simulink model "xieboduoji_13fangzhennow"  (R2023a)
settings: Solver=ode4  StartTime=0.0  StopTime=2.2  FixedStep=5e-7  RelTol=1e-3
undefined symbols (not defined in the file or in its folder): magnitude
libraries: simulink x417, spsRMSLib x70, spsCurrentMeasurementLib x32, spsVoltageMeasurementLib x31, powerlib_meascontrol x24, spsFourierLib x21, spsGroundLib x19, spsThreePhasePISectionLineLib x17, spsThreePhaseSeriesRLCBranchLib x14, spsdq0toAlphaBetaZeroLib x13, spsSeriesRLCBranchLib x11, spsUniversalBridgeLib x11
(part 4 of 12)

== system xieboduoji_13fangzhennow/node14/PV15kW3/Subsystem9 ==
  di : Inport
  Enable : EnablePort
  Pulse tor2 : DiscretePulseGenerator  PulseType=Time based  Period=10e-5  PulseWidth=50
  "integral " : Subsystem  TreatAsAtomicUnit=on
  w : Outport
  wires:
  Pulse tor2/1 -> "integral "/Trigger
  di/1 -> "integral "/1(di)
  "integral "/1(w) -> w/1

== system xieboduoji_13fangzhennow/node14/PV15kW3/改进PLL1 ==
  abc : Inport
  Add : Sum
  Alpha-Beta-Zero to dq0 : spsAlphaBetaZerotodq0Lib/Alpha-Beta-Zero to dq0  Alignment=Aligned with phase A axis
  Constant : Constant  Value=100*pi
  Constant3 : Constant  Value=2*pi
  Demux1 : Demux  Outputs=3
  Gain1 : Gain  Commented=on  Gain=0.5/pi
  Goto2 : Goto  Commented=on  GotoTag=vp
  Integrator : Integrator
  Math Function : Math  Operator=mod  SignedPower=on
  PI : Subsystem  TreatAsAtomicUnit=on
  PID Controller : slpidlib/PID Controller  Controller=P  Form=Parallel  TimeDomain=Discrete-time  UseExternalTs=off  SampleTime=10e-5  IntegratorMethod=Forward Euler  FilterMethod=Forward Euler  ControllerParametersSource=internal  P=1  I=1  UseKiTs=off  D=0  N=100  UseFilter=on  TunerSelectOption=Transfer Function Based (PID Tuner App)  InitialConditionSource=internal  InitialConditionForIntegrator=0  InitialConditionForFilter=0  DifferentiatorICPrevScaledInput=0  ExternalReset=none  TrackingMode=off  Kt=1  LimitOutput=off  SatLimitsSource=internal  UpperSaturationLimit=inf  LowerSaturationLimit=-inf  LinearizeAsGain=on  AntiWindupMode=none  Kb=1  LimitIntegrator=off  UpperIntegratorSaturationLimit=inf  LowerIntegratorSaturationLimit=-inf  POutMin=[]  POutMax=[]  IOutMin=[]  IOutMax=[]  DOutMin=[]  DOutMax=[]  NOutMin=[]  NOutMax=[]  SumOutMin=[]  SumOutMax=[]  SaturationOutMin=[]  SaturationOutMax=[]  PParamMin=[]  PParamMax=[]  IParamMin=[]  IParamMax=[]  DParamMin=[]  DParamMax=[]  NParamMin=[]  NParamMax=[]  KbParamMin=[]  KbParamMax=[]  KtParamMin=[]  KtParamMax=[]  KbOutMin=[]  KbOutMax=[]  KtOutMin=[]  KtOutMax=[]  IntegratorOutMin=[]  IntegratorOutMax=[]  FilterOutMin=[]  FilterOutMax=[]  SumI1OutMin=[]  SumI1OutMax=[]  SumI2OutMin=[]  SumI2OutMax=[]  SumI3OutMin=[]  SumI3OutMax=[]  SumI4OutMin=[]  SumI4OutMax=[]  SumDOutMin=[]  SumDOutMax=[]  DifferentiatorOutMin=[]  DifferentiatorOutMax=[]  FilterDiffOutCoefMin=[]  FilterDiffOutCoefMax=[]  ReciprocalOutMin=[]  ReciprocalOutMax=[]  SumDenOutMin=[]  SumDenOutMax=[]  SumNumOutMin=[]  SumNumOutMax=[]  DivideOutMin=[]  DivideOutMax=[]  UdiffTsProdOutMin=[]  UdiffTsProdOutMax=[]  NTsProdOutMin=[]  NTsProdOutMax=[]  UintegralTsProdOutMin=[]  UintegralTsProdOutMax=[]  UngainTsProdOutMin=[]  UngainTsProdOutMax=[]  ClampingZeroOutDataTypeStr=Inherit: Inherit via back propagation  ClampingZeroOutMin=[]  ClampingZeroOutMax=[]  FilterDenConstantOutDataTypeStr=Inherit: Inherit via back propagation  FilterDenConstantOutMin=[]  FilterDenConstantOutMax=[]  PCopyOutDataTypeStr=Inherit: Inherit via back propagation  PCopyOutMin=[]  PCopyOutMax=[]  NCopyOutDataTypeStr=Inherit: Inherit via back propagation  NCopyOutMin=[]  NCopyOutMax=[]  IntegratorContinuousStateAttributes=''  IntegratorStateMustResolveToSignalObject=off  IntegratorRTWStateStorageClass=Auto  FilterContinuousStateAttributes=''  FilterStateMustResolveToSignalObject=off  FilterRTWStateStorageClass=Auto  ParallelPVariant=InternalParameters  IdealPVariant=Disabled  IVariant=Disabled  DVariant=Disabled  IntegratorVariant=Disabled  SatVariant=Disabled  AWVariant=Disabled  PCopyVariant=Disabled  TRVariant=Disabled  FdbkBlocksVariant=Forward  IdealPFdbkVariant=Disabled  SatFdbkVariant=Disabled  DerivativeFilterVariant=Disabled  NVariant=Disabled  NCopyVariant=Disabled_SignalSpec  FilterICVariant=Disabled  IntegratorICVariant=Disabled  ExternalResetVariant=Disabled  TRSumVariant=Passthrough  SumFdbkVariant=Disabled  SumVariant=Passthrough_P  TsampFilterVariant=InternalTs  TsampNgainVariant=Passthrough  TsampIntegralVariant=Disabled_SignalSpec  ExternalSaturationOutDataTypeStr=Inherit: Same as second input
  Pulse tor2 : DiscretePulseGenerator  PulseType=Time based  Period=5e-5  PulseWidth=50
  Scope : Scope
  Scope1 : Scope  Commented=on
  Scope3 : Scope  Commented=on
  Subsystem2 : Subsystem
  Terminator : Terminator
  abc to Alpha-Beta-Zero1 : spsabctoAlphaBetaZeroLib/abc to Alpha-Beta-Zero
  mean1 : spsMeanLib/Mean  Commented=on  Freq=100  Vinit=0  Ts=10e-5
  mean2 : spsMeanLib/Mean  Freq=100  Vinit=0  Ts=10e-5
  Out2 : Outport
  vab0 : Outport  Port=2
  wires:
  Demux1/3 -> Terminator/1
  mean2/1 -> PID Controller/1, PI/1(Vgq)
  abc/1 -> abc to Alpha-Beta-Zero1/1
  mean1/1 -> Scope3/1, Goto2/1
  Demux1/2 -> mean2/1
  Pulse tor2/1 -> PI/Trigger
  PI/1(w) -> Add/2
  Constant/1 -> Add/1
  Alpha-Beta-Zero to dq0/1 -> Demux1/1
  Add/1 -> Gain1/1, Integrator/1
  Math Function/1 -> Out2/1, [wt], Alpha-Beta-Zero to dq0/2
  Constant3/1 -> Math Function/2
  Integrator/1 -> Math Function/1
  Gain1/1 -> Scope1/1
  PID Controller/1 -> Scope/1
  Demux1/1 -> mean1/1
  abc to Alpha-Beta-Zero1/1 -> vab0/1, Subsystem2/1(In1)
  Subsystem2/1(Out1) -> Alpha-Beta-Zero to dq0/1

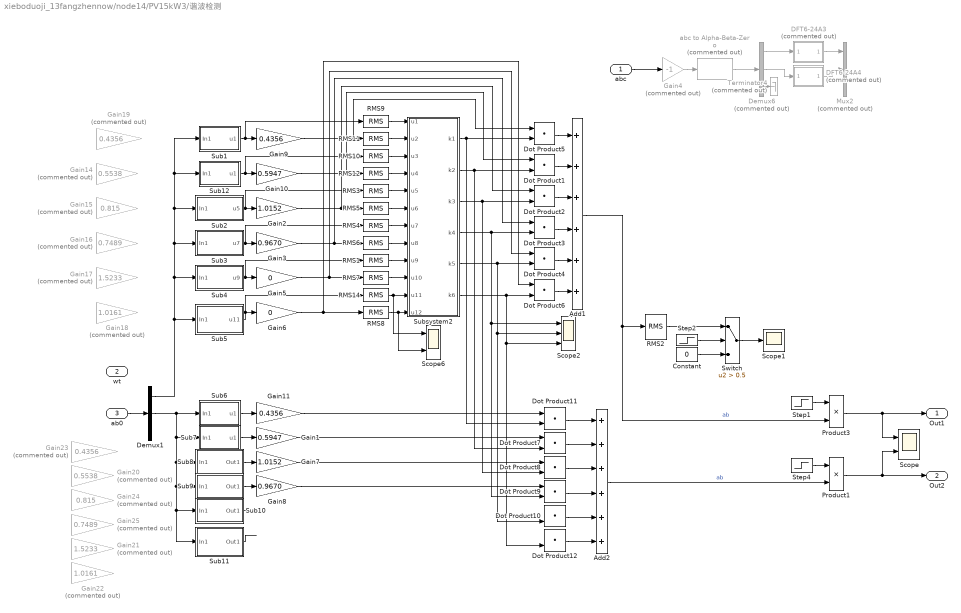
== system xieboduoji_13fangzhennow/node14/PV15kW3/谐波检测 ==
  abc : Inport
  wt : Inport  Port=2
  ab0 : Inport  Port=3
  Add1 : Sum  Inputs=++++++
  Add2 : Sum  Inputs=++++++
  Constant : Constant  Value=0
  DFT6-24A3 : Subsystem  Commented=on
  DFT6-24A4 : Subsystem  Commented=on
  Demux1 : Demux  Outputs=3
  Demux6 : Demux  Commented=on  Outputs=3
  Dot Product{1..12} (12 alike) : DotProduct  OutDataTypeStr=Inherit: Inherit via internal rule
  Gain1 : Gain  Gain=0.5947
  Gain10 : Gain  Gain=0.5947
  Gain11 : Gain  Gain=0.4356
  Gain14 : Gain  Commented=on  Gain=0.5538
  Gain15 : Gain  Commented=on  Gain=0.815
  Gain16 : Gain  Commented=on  Gain=0.7489
  Gain17 : Gain  Commented=on  Gain=1.5233
  Gain18 : Gain  Commented=on  Gain=1.0161
  Gain19 : Gain  Commented=on  Gain=0.4356
  Gain2 : Gain  Gain=1.0152
  Gain20 : Gain  Commented=on  Gain=0.5538
  Gain21 : Gain  Commented=on  Gain=1.5233
  Gain22 : Gain  Commented=on  Gain=1.0161
  Gain23 : Gain  Commented=on  Gain=0.4356
  Gain24 : Gain  Commented=on  Gain=0.815
  Gain25 : Gain  Commented=on  Gain=0.7489
  Gain3 : Gain  Gain=0.9670
  Gain4 : Gain  Commented=on  Gain=-1
  Gain5 : Gain  Gain=0
  Gain6 : Gain  Gain=0
  Gain7 : Gain  Gain=1.0152
  Gain8 : Gain  Gain=0.9670
  Gain9 : Gain  Gain=0.4356
  Mux2 : Mux  Commented=on  Inputs=3
  Product1 : Product
  Product3 : Product
  RMS{1,3..12,14} (12 alike) : spsRMSLib/RMS  TrueRMS=on  Freq=100  RMSInit=0  Ts=5e-5
  RMS2 : spsRMSLib/RMS  TrueRMS=on  Freq=50  RMSInit=0  Ts=5e-5
  Scope : Scope  NumInputPorts=2
  Scope1 : Scope
  Scope2 : Scope  NumInputPorts=3
  Scope6 : Scope  NumInputPorts=2
  Step1 : Step  After=-1  SampleTime=0
  Step2 : Step  SampleTime=0
  Step4 : Step  After=-1  SampleTime=0
  Sub1 : Subsystem
  Sub10 : Subsystem
  Sub11 : Subsystem
  Sub12 : Subsystem
  Sub2 : Subsystem
  Sub3 : Subsystem
  Sub4 : Subsystem
  Sub5 : Subsystem
  Sub6 : Subsystem
  Sub7 : Subsystem
  Sub8 : Subsystem
  Sub9 : Subsystem
  Subsystem2 : Subsystem
  Switch : Switch  Criteria=u2 > Threshold  Threshold=0.5  SaturateOnIntegerOverflow=off  InputSameDT=off
  Terminator4 : Terminator  Commented=on
  abc to Alpha-Beta-Zero : spsabctoAlphaBetaZeroLib/abc to Alpha-Beta-Zero  Commented=on
  Out1 : Outport
  Out2 : Outport  Port=2
  wires:
  abc/1 -> Gain4/1
  Step1/1 -> Product3/1
  abc to Alpha-Beta-Zero/1 -> Demux6/1
  DFT6-24A4/1(Out1) -> Mux2/2
  DFT6-24A3/1(Out1) -> Mux2/1
  Demux6/2 -> DFT6-24A4/1(In1)
  Demux6/1 -> DFT6-24A3/1(In1)
  Demux6/3 -> Terminator4/1
  ab0/1 -> Demux1/1
  Step2/1 -> Switch/2
  Constant/1 -> Switch/3
  Switch/1 -> Scope1/1
  Gain4/1 -> abc to Alpha-Beta-Zero/1
  Sub5/1(u11) -> RMS14/1, Gain6/1
  Sub4/1(u9) -> Gain5/1, RMS1/1
  Sub3/1(u7) -> RMS4/1, Gain3/1
  Sub2/1(u5) -> RMS3/1, Gain2/1
  Demux1/1 -> Sub12/1(In1), Sub1/1(In1), Sub2/1(In1), Sub3/1(In1), Sub4/1(In1), Sub5/1(In1)
  Sub12/1(u1) -> RMS10/1, Gain10/1
  Sub1/1(u1) -> RMS9/1, Gain9/1
  Subsystem2/1(k1) -> Dot Product11/2, Dot Product5/2
  Subsystem2/2(k2) -> Dot Product7/2, Dot Product1/2
  Subsystem2/3(k3) -> Dot Product8/2, Dot Product2/2
  Subsystem2/4(k4) -> Scope2/1, Dot Product9/2, Dot Product3/2
  Subsystem2/5(k5) -> Dot Product10/2, Scope2/2, Dot Product4/2
  Add1/1 -> Product3/2, RMS2/1  "ab"
  Sub6/1(u1) -> Gain11/1
  Sub7/1(u1) -> Gain1/1
  Sub8/1(Out1) -> Gain7/1
  Sub9/1(Out1) -> Gain8/1
  Sub10/1(Out1) -> ?
  Sub11/1(Out1) -> ?
  Demux1/2 -> Sub6/1(In1), Sub7/1(In1), Sub11/1(In1), Sub10/1(In1), Sub9/1(In1), Sub8/1(In1)
  Dot Product12/1 -> Add2/6
  Dot Product10/1 -> Add2/5
  Gain9/1 -> RMS11/1, Dot Product5/1
  Gain2/1 -> RMS5/1, Dot Product2/1
  Gain3/1 -> Dot Product3/1, RMS6/1
  Gain5/1 -> RMS7/1, Dot Product4/1
  Gain6/1 -> Dot Product6/1, RMS8/1
  Gain11/1 -> Dot Product11/1
  Gain1/1 -> Dot Product7/1
  Gain7/1 -> Dot Product8/1
  Gain8/1 -> Dot Product9/1
  ? -> Dot Product10/1
  ? -> Dot Product12/1
  RMS2/1 -> Switch/1
  RMS7/1 -> Subsystem2/10(u10)
  RMS8/1 -> Scope6/2, Subsystem2/12(u12)
  Gain10/1 -> RMS12/1, Dot Product1/1
  RMS9/1 -> Subsystem2/1(u1)
  RMS1/1 -> Subsystem2/9(u9)
  RMS14/1 -> Subsystem2/11(u11), Scope6/1
  Dot Product6/1 -> Add1/6
  Dot Product4/1 -> Add1/5
  RMS11/1 -> Subsystem2/2(u2)
  RMS10/1 -> Subsystem2/3(u3)
  RMS12/1 -> Subsystem2/4(u4)
  RMS3/1 -> Subsystem2/5(u5)
  RMS5/1 -> Subsystem2/6(u6)
  RMS4/1 -> Subsystem2/7(u7)
  RMS6/1 -> Subsystem2/8(u8)
  Add2/1 -> Product1/2  "ab"
  Step4/1 -> Product1/1
  Product1/1 -> Scope/2, Out2/1
  Product3/1 -> Scope/1, Out1/1
  Dot Product5/1 -> Add1/1
  Dot Product1/1 -> Add1/2
  Dot Product2/1 -> Add1/3
  Dot Product3/1 -> Add1/4
  Subsystem2/6(k6) -> Scope2/3, Dot Product12/2, Dot Product6/2
  Dot Product11/1 -> Add2/1
  Dot Product7/1 -> Add2/2
  Dot Product8/1 -> Add2/3
  Dot Product9/1 -> Add2/4

== system xieboduoji_13fangzhennow/node14/Subsystem1/RMS1 ==
  u1 : Inport
  u3 : Inport  Port=2
  u4 : Inport  Port=3
  u5 : Inport  Port=4
  u6 : Inport  Port=5
  u2 : Inport  Port=6
  Trigger : TriggerPort  VariantControl=(inherit)
  Scope : Scope  Commented=on
  Scope1 : Scope  Commented=on
  xunidiandao : MATLAB Function  TreatAsAtomicUnit=on
  k1 : Outport  VectorParamsAs1DForOutWhenUnconnected=off
  k2 : Outport  Port=2  VectorParamsAs1DForOutWhenUnconnected=off
  k3 : Outport  Port=3  VectorParamsAs1DForOutWhenUnconnected=off
  k4 : Outport  Port=4  VectorParamsAs1DForOutWhenUnconnected=off
  k5 : Outport  Port=5  VectorParamsAs1DForOutWhenUnconnected=off
  k6 : Outport  Port=6  VectorParamsAs1DForOutWhenUnconnected=off
  k7 : Outport  Port=7  VectorParamsAs1DForOutWhenUnconnected=off
  k8 : Outport  Port=8  VectorParamsAs1DForOutWhenUnconnected=off
  k9 : Outport  Port=9  VectorParamsAs1DForOutWhenUnconnected=off
  k10 : Outport  Port=10  VectorParamsAs1DForOutWhenUnconnected=off
  k11 : Outport  Port=11  VectorParamsAs1DForOutWhenUnconnected=off
  k12 : Outport  Port=12  VectorParamsAs1DForOutWhenUnconnected=off
  wires:
  xunidiandao/13(x) -> Scope/1
  u3/1 -> xunidiandao/2(u2)
  u4/1 -> xunidiandao/3(u3)
  u5/1 -> xunidiandao/4(u4)
  u6/1 -> xunidiandao/5(u5)
  u2/1 -> xunidiandao/6(u6)
  u1/1 -> xunidiandao/1(u1)
  xunidiandao/12(y66) -> k12/1
  xunidiandao/11(y6) -> k11/1
  xunidiandao/10(y55) -> k10/1
  xunidiandao/9(y5) -> k9/1
  xunidiandao/8(y44) -> k8/1
  xunidiandao/7(y4) -> k7/1
  xunidiandao/6(y33) -> k6/1
  xunidiandao/5(y3) -> k5/1
  xunidiandao/4(y22) -> k4/1
  xunidiandao/3(y2) -> k3/1
  xunidiandao/2(y11) -> k2/1
  xunidiandao/1(y1) -> k1/1, Scope1/1

== system xieboduoji_13fangzhennow/node14/Subsystem2/RMS1 ==
  u1 : Inport
  u3 : Inport  Port=2
  u4 : Inport  Port=3
  u5 : Inport  Port=4
  u6 : Inport  Port=5
  u2 : Inport  Port=6
  Trigger : TriggerPort  VariantControl=(inherit)
  Scope : Scope  Commented=on
  Scope1 : Scope  Commented=on
  xunidiandao : MATLAB Function  TreatAsAtomicUnit=on
  k1 : Outport  VectorParamsAs1DForOutWhenUnconnected=off
  k2 : Outport  Port=2  VectorParamsAs1DForOutWhenUnconnected=off
  k3 : Outport  Port=3  VectorParamsAs1DForOutWhenUnconnected=off
  k4 : Outport  Port=4  VectorParamsAs1DForOutWhenUnconnected=off
  k5 : Outport  Port=5  VectorParamsAs1DForOutWhenUnconnected=off
  k6 : Outport  Port=6  VectorParamsAs1DForOutWhenUnconnected=off
  k7 : Outport  Port=7  VectorParamsAs1DForOutWhenUnconnected=off
  k8 : Outport  Port=8  VectorParamsAs1DForOutWhenUnconnected=off
  k9 : Outport  Port=9  VectorParamsAs1DForOutWhenUnconnected=off
  k10 : Outport  Port=10  VectorParamsAs1DForOutWhenUnconnected=off
  k11 : Outport  Port=11  VectorParamsAs1DForOutWhenUnconnected=off
  k12 : Outport  Port=12  VectorParamsAs1DForOutWhenUnconnected=off
  wires:
  xunidiandao/1(y1) -> Scope1/1, k1/1
  xunidiandao/2(y11) -> k2/1
  xunidiandao/3(y2) -> k3/1
  xunidiandao/4(y22) -> k4/1
  xunidiandao/5(y3) -> k5/1
  xunidiandao/6(y33) -> k6/1
  xunidiandao/7(y4) -> k7/1
  xunidiandao/8(y44) -> k8/1
  xunidiandao/9(y5) -> k9/1
  xunidiandao/10(y55) -> k10/1
  xunidiandao/11(y6) -> k11/1
  xunidiandao/12(y66) -> k12/1
  u1/1 -> xunidiandao/1(u1)
  u2/1 -> xunidiandao/6(u6)
  u6/1 -> xunidiandao/5(u5)
  u5/1 -> xunidiandao/4(u4)
  u4/1 -> xunidiandao/3(u3)
  u3/1 -> xunidiandao/2(u2)
  xunidiandao/13(x) -> Scope/1

== system xieboduoji_13fangzhennow/node14/谐波源/Subsystem1 ==
  u1 : Inport
  u3 : Inport  Port=2
  u4 : Inport  Port=3
  u5 : Inport  Port=4
  u6 : Inport  Port=5
  u2 : Inport  Port=6
  Pul : DiscretePulseGenerator  PulseType=Time based  Period=5e-5  PulseWidth=40
  RMS1 : Subsystem  TreatAsAtomicUnit=on
  k1 : Outport  VectorParamsAs1DForOutWhenUnconnected=off
  k2 : Outport  Port=2  VectorParamsAs1DForOutWhenUnconnected=off
  k3 : Outport  Port=3  VectorParamsAs1DForOutWhenUnconnected=off
  k4 : Outport  Port=4  VectorParamsAs1DForOutWhenUnconnected=off
  k5 : Outport  Port=5  VectorParamsAs1DForOutWhenUnconnected=off
  k6 : Outport  Port=6  VectorParamsAs1DForOutWhenUnconnected=off
  k7 : Outport  Port=7  VectorParamsAs1DForOutWhenUnconnected=off
  k8 : Outport  Port=8  VectorParamsAs1DForOutWhenUnconnected=off
  k9 : Outport  Port=9  VectorParamsAs1DForOutWhenUnconnected=off
  k10 : Outport  Port=10  VectorParamsAs1DForOutWhenUnconnected=off
  k11 : Outport  Port=11  VectorParamsAs1DForOutWhenUnconnected=off
  k12 : Outport  Port=12  VectorParamsAs1DForOutWhenUnconnected=off
  wires:
  u2/1 -> RMS1/6(u2)
  u6/1 -> RMS1/5(u6)
  u5/1 -> RMS1/4(u5)
  u4/1 -> RMS1/3(u4)
  u3/1 -> RMS1/2(u3)
  u1/1 -> RMS1/1(u1)
  RMS1/12(k12) -> k12/1
  RMS1/11(k11) -> k11/1
  RMS1/10(k10) -> k10/1
  RMS1/9(k9) -> k9/1
  RMS1/8(k8) -> k8/1
  RMS1/7(k7) -> k7/1
  RMS1/6(k6) -> k6/1
  RMS1/5(k5) -> k5/1
  RMS1/4(k4) -> k4/1
  RMS1/3(k3) -> k3/1
  RMS1/2(k2) -> k2/1
  RMS1/1(k1) -> k1/1
  Pul/1 -> RMS1/Trigger

== system xieboduoji_13fangzhennow/node14/谐波源/Subsystem2 ==
  u1 : Inport
  u3 : Inport  Port=2
  u4 : Inport  Port=3
  u5 : Inport  Port=4
  u6 : Inport  Port=5
  u2 : Inport  Port=6
  Pul : DiscretePulseGenerator  PulseType=Time based  Period=5e-5  PulseWidth=40
  RMS1 : Subsystem  TreatAsAtomicUnit=on
  k1 : Outport  VectorParamsAs1DForOutWhenUnconnected=off
  k2 : Outport  Port=2  VectorParamsAs1DForOutWhenUnconnected=off
  k3 : Outport  Port=3  VectorParamsAs1DForOutWhenUnconnected=off
  k4 : Outport  Port=4  VectorParamsAs1DForOutWhenUnconnected=off
  k5 : Outport  Port=5  VectorParamsAs1DForOutWhenUnconnected=off
  k6 : Outport  Port=6  VectorParamsAs1DForOutWhenUnconnected=off
  k7 : Outport  Port=7  VectorParamsAs1DForOutWhenUnconnected=off
  k8 : Outport  Port=8  VectorParamsAs1DForOutWhenUnconnected=off
  k9 : Outport  Port=9  VectorParamsAs1DForOutWhenUnconnected=off
  k10 : Outport  Port=10  VectorParamsAs1DForOutWhenUnconnected=off
  k11 : Outport  Port=11  VectorParamsAs1DForOutWhenUnconnected=off
  k12 : Outport  Port=12  VectorParamsAs1DForOutWhenUnconnected=off
  wires:
  Pul/1 -> RMS1/Trigger
  RMS1/1(k1) -> k1/1
  RMS1/2(k2) -> k2/1
  RMS1/3(k3) -> k3/1
  RMS1/4(k4) -> k4/1
  RMS1/5(k5) -> k5/1
  RMS1/6(k6) -> k6/1
  RMS1/7(k7) -> k7/1
  RMS1/8(k8) -> k8/1
  RMS1/9(k9) -> k9/1
  RMS1/10(k10) -> k10/1
  RMS1/11(k11) -> k11/1
  RMS1/12(k12) -> k12/1
  u1/1 -> RMS1/1(u1)
  u3/1 -> RMS1/2(u3)
  u4/1 -> RMS1/3(u4)
  u5/1 -> RMS1/4(u5)
  u6/1 -> RMS1/5(u6)
  u2/1 -> RMS1/6(u2)

== system xieboduoji_13fangzhennow/node3/PV15kW2/PV_Cells2 ==
  note: I0
  note: Iph
  G : Inport
  T : Inport  Port=2
  U : Inport  Port=3
  Add{,3..4,6} (4 alike) : Sum
  Add1 : Sum  Inputs=+-
  Add2 : Sum  Inputs=-+
  Add5 : Sum  Inputs=-+
  Add7 : Sum  Inputs=+-
  C to K : Constant  Value=273.16
  Controlled Current Source : spsControlledCurrentSourceLib/Controlled Current Source  Initialize=on  Source_Type=DC  Amplitude=0  Phase=0  Frequency=0  Measurements=None
  Current Measurement : spsCurrentMeasurementLib/Current Measurement  PhasorSimulation=off  OutputType=Complex  PSBequivalent=0
  Divide{,1..3} (4 alike) : Product  Inputs=*/
  Divide4 : Product  Inputs=**
  Gain : Gain  Gain=1/Series
  Gain1 : Gain  Gain=1/Parallel
  Gn : Constant  Value=1000
  Isc,n : Constant  Value=8.214*Parallel
  Ki : Constant  Value=0.0032*Parallel
  Kv : Constant  Value=-0.123
  Math : Math  SignedPower=on
  Math2 : Math  SignedPower=on
  Nc*K/Q*a : Constant  Value=0.00008629*1.3*54
  Product{,1..4} (5 alike) : Product  RndMeth=Zero
  Rs : Constant  Value=0.221
  Scope : Scope
  Tn : Constant  Value=298.16
  Unit Delay : UnitDelay  SampleTime=-1  HasFrameUpgradeWarning=on
  Voc,n : Constant  Value=32.9
  constant : Constant
  constant2 : Constant
  I_positive : PMIOPort  Tag=PMCPort  Side=Right
  I_negative : PMIOPort  Tag=PMCPort  Port=2  Side=Right
  wires:
  Divide4/1 -> Add6/2  "Rs"
  Divide/1 -> Product/1
  Isc,n/1 -> Add/1
  Product1/1 -> Add/2
  Divide2/1 -> Math/1
  Add/1 -> [I], Product/2
  T/1 -> Add3/1
  Add2/1 -> Divide1/2
  Math/1 -> Add2/2
  [I] -> Divide1/1
  Add1/1 -> [delta_T], Product1/1
  Tn/1 -> Add1/2
  Ki/1 -> Product1/2
  Product/1 -> Add7/1
  Nc*K/Q*a/1 -> Product2/2
  Kv/1 -> Product3/1
  Voc,n/1 -> Add4/2
  Current Measurement/1 -> Unit Delay/1
  [T] -> Product2/1
  [delta_T] -> Product3/2
  Add6/1 -> Divide3/1
  U/1 -> Gain/1
  Rs/1 -> Divide4/1
  Divide1/1 -> Product4/1
  Add7/1 -> Controlled Current Source/1
  Product4/1 -> Add7/2
  constant2/1 -> Add5/1
  Add5/1 -> Product4/2
  [Iout] -> Gain1/1
  Math2/1 -> Scope/1, Add5/2
  Divide3/1 -> Math2/1
  C to K/1 -> Add3/2
  Product2/1 -> Divide3/2, Divide2/2  "Vt*a"
  Add4/1 -> Divide2/1
  Product3/1 -> Add4/1
  Gn/1 -> Divide/2
  constant/1 -> Add2/1
  Add3/1 -> [T], Add1/1
  G/1 -> Divide/1
  Unit Delay/1 -> [Iout]
  Gain/1 -> Add6/1
  Gain1/1 -> Divide4/2
  connections:
  I_negative/RConn1 -- Controlled Current Source/LConn1
  I_positive/RConn1 -- Current Measurement/RConn1
  Controlled Current Source/RConn1 -- Current Measurement/LConn1

== system xieboduoji_13fangzhennow/node3/PV15kW2/PWM2 ==
  Via* : Inport
  Vib* : Inport  Port=2
  Enable : EnablePort
  Alpha-Beta-Zero to abc1 : powerlib_meascontrol/Transformations/Alpha-Beta-Zero to abc
  Mux1 : Mux  Inputs=3
  PWM3 : Subsystem
  Transport Delay2 : TransportDelay  DelayTime=5e-5
  switch : Outport  PortDimensions=6  VectorParamsAs1DForOutWhenUnconnected=off
  Out1 : Outport  Port=2  VectorParamsAs1DForOutWhenUnconnected=off
  wires:
  Via*/1 -> Mux1/1
  Vib*/1 -> Mux1/2
  Alpha-Beta-Zero to abc1/1 -> PWM3/1(In1)
  PWM3/1(switch) -> switch/1
  PWM3/2(Out1) -> Out1/1
  Mux1/1 -> Transport Delay2/1
  Transport Delay2/1 -> Alpha-Beta-Zero to abc1/1

== system xieboduoji_13fangzhennow/node3/PV15kW2/Subsystem3 ==
  In2 : Inport
  In1 : Inport  Port=2
  Add1 : Sum  Inputs=+++
  Add3 : Sum  Inputs=+++
  Demux{1..3,5} (4 alike) : Demux  Outputs=3
  Mux1 : Mux  Inputs=3
  Mux2 : Mux  Inputs=3
  Mux3 : Mux  Inputs=3
  Terminator : Terminator
  Transfer Fcn1 : TransferFcn  Numerator=[3.2*3.14 0]  Denominator=[1 0.7*3.14 360000*pi*pi]
  Transfer Fcn10 : TransferFcn  Commented=on  Numerator=[1.7*3.14*0.766 -1.7*3.14*1200*pi*0.643]  Denominator=[1 0.6*3.14 1440000*pi*pi]
  Transfer Fcn11 : TransferFcn  Commented=on  Numerator=[1*3.14*0.5 -1*3.14*1800*pi*0.866]  Denominator=[1 0.4*3.14 3240000*pi*pi]
  Transfer Fcn12 : TransferFcn  Commented=on  Numerator=[1.2*3.14*0.5 -1.2*3.14*1800*pi*0.866]  Denominator=[1 0.4*3.14 3240000*pi*pi]
  Transfer Fcn13 : TransferFcn  Commented=on  Numerator=[1.2*3.14*0.1736 -1.2*3.14*1800*pi*0.9848]  Denominator=[1 0.4*3.14 3240000*pi*pi]
  Transfer Fcn17 : TransferFcn  Commented=on  Numerator=[1.9*3.14*0.766 -1.9*3.14*1200*pi*0.643]  Denominator=[1 0.6*3.14 1440000*pi*pi]
  Transfer Fcn18 : TransferFcn  Commented=on  Numerator=[1.2*3.14*0.5 -1.2*3.14*1800*pi*0.866]  Denominator=[1 0.4*3.14 3240000*pi*pi]
  Transfer Fcn19 : TransferFcn  Commented=on  Numerator=[1.9*3.14*0.9703 -1.9*3.14*1200*pi*0.2419]  Denominator=[1 0.55*3.14 1440000*pi*pi]
  Transfer Fcn2 : TransferFcn  Numerator=[1.9*3.14*0.866 -1.9*3.14*1200*pi*0.5]  Denominator=[1 0.55*3.14 1440000*pi*pi]
  Transfer Fcn3 : TransferFcn  Numerator=[1.2*3.14*0.707 -1.2*3.14*1800*pi*0.707]  Denominator=[1 0.4*3.14 3240000*pi*pi]
  Transfer Fcn4 : TransferFcn  Numerator=[3.2*3.14 0]  Denominator=[1 0.7*3.14 360000*pi*pi]
  Transfer Fcn5 : TransferFcn  Commented=on  Numerator=[2.4*3.14 0]  Denominator=[1 0.8*3.14 360000*pi*pi]
  Transfer Fcn6 : TransferFcn  Numerator=[1.2*3.14*0.707 -1.2*3.14*1800*pi*0.707]  Denominator=[1 0.4*3.14 3240000*pi*pi]
  Transfer Fcn7 : TransferFcn  Commented=on  Numerator=[1.9*3.14*0.766 -1.9*3.14*1200*pi*0.643]  Denominator=[1 0.55*3.14 1440000*pi*pi]
  Transfer Fcn8 : TransferFcn  Numerator=[1.9*3.14*0.866 -1.9*3.14*1200*pi*0.5]  Denominator=[1 0.55*3.14 1440000*pi*pi]
  Transfer Fcn9 : TransferFcn  Commented=on  Numerator=[3*3.14 0]  Denominator=[1 0.7*3.14 360000*pi*pi]
  dq0 to Alpha-Beta-Zero : powerlib_meascontrol/Transformations/dq0 to Alpha-Beta-Zero  Alignment=90 degrees behind phase A axis
  dq0 to Alpha-Beta-Zero1 : powerlib_meascontrol/Transformations/dq0 to Alpha-Beta-Zero  Alignment=90 degrees behind phase A axis
  dq0 to Alpha-Beta-Zero2 : powerlib_meascontrol/Transformations/dq0 to Alpha-Beta-Zero  Alignment=90 degrees behind phase A axis
  Out3 : Outport
  Out1 : Outport  Port=2
  wires:
  In2/1 -> Demux5/1
  Demux5/1 -> Transfer Fcn2/1, Transfer Fcn3/1, Transfer Fcn4/1
  Transfer Fcn4/1 -> Mux1/1
  Transfer Fcn1/1 -> Mux1/2
  Mux1/1 -> dq0 to Alpha-Beta-Zero/1
  dq0 to Alpha-Beta-Zero/1 -> Demux1/1
  Demux1/1 -> Add1/1
  Demux1/2 -> Add3/1
  Add1/1 -> Out3/1
  Add3/1 -> Out1/1
  dq0 to Alpha-Beta-Zero1/1 -> Demux2/1
  Mux2/1 -> dq0 to Alpha-Beta-Zero1/1
  Transfer Fcn8/1 -> Mux2/2
  Transfer Fcn2/1 -> Mux2/1
  Demux2/1 -> Add1/2
  Demux2/2 -> Add3/2
  Demux3/2 -> Add3/3
  Demux3/1 -> Add1/3
  Transfer Fcn3/1 -> Mux3/1
  Transfer Fcn6/1 -> Mux3/2
  Mux3/1 -> dq0 to Alpha-Beta-Zero2/1
  dq0 to Alpha-Beta-Zero2/1 -> Demux3/1
  Demux5/2 -> Transfer Fcn1/1, Transfer Fcn8/1, Transfer Fcn6/1
  In1/1 -> dq0 to Alpha-Beta-Zero1/2, dq0 to Alpha-Beta-Zero2/2, dq0 to Alpha-Beta-Zero/2
  Demux5/3 -> Terminator/1

== system xieboduoji_13fangzhennow/node3/PV15kW2/Subsystem7 ==
  Voltage : spsVoltageMeasurementLib/Voltage Measurement  PhasorSimulation=off  OutputType=Complex  PSBequivalent=0
  Voltage1 : spsVoltageMeasurementLib/Voltage Measurement  PhasorSimulation=off  OutputType=Complex  PSBequivalent=0
  Voltage2 : spsVoltageMeasurementLib/Voltage Measurement  PhasorSimulation=off  OutputType=Complex  PSBequivalent=0
  1 : PMIOPort  Side=Left
  2 : PMIOPort  Port=2  Side=Left
  3 : PMIOPort  Port=3  Side=Left
  4 : PMIOPort  Port=4  Side=Left
  5 : PMIOPort  Port=5  Side=Left
  6 : PMIOPort  Port=6  Side=Left
  O1 : Outport  VectorParamsAs1DForOutWhenUnconnected=off
  O2 : Outport  Port=2  VectorParamsAs1DForOutWhenUnconnected=off
  O3 : Outport  Port=3  VectorParamsAs1DForOutWhenUnconnected=off
  wires:
  Voltage2/1 -> O3/1
  Voltage1/1 -> O2/1
  Voltage/1 -> O1/1
  connections:
  6/RConn1 -- Voltage2/LConn2
  5/RConn1 -- Voltage2/LConn1
  4/RConn1 -- Voltage1/LConn2
  3/RConn1 -- Voltage1/LConn1
  2/RConn1 -- Voltage/LConn2
  1/RConn1 -- Voltage/LConn1

== system xieboduoji_13fangzhennow/node3/PV15kW2/Subsystem8 ==
  Current : spsCurrentMeasurementLib/Current Measurement  PhasorSimulation=off  OutputType=Complex  PSBequivalent=0
  Current 2 : spsCurrentMeasurementLib/Current Measurement  PhasorSimulation=off  OutputType=Complex  PSBequivalent=0
  Current1 : spsCurrentMeasurementLib/Current Measurement  PhasorSimulation=off  OutputType=Complex  PSBequivalent=0
  1 : PMIOPort  Side=Left
  2 : PMIOPort  Port=2  Side=Right
  3 : PMIOPort  Port=3  Side=Left
  4 : PMIOPort  Port=4  Side=Right
  5 : PMIOPort  Port=5  Side=Left
  6 : PMIOPort  Port=6  Side=Right
  O1 : Outport  VectorParamsAs1DForOutWhenUnconnected=off
  O2 : Outport  Port=2  VectorParamsAs1DForOutWhenUnconnected=off
  O3 : Outport  Port=3  VectorParamsAs1DForOutWhenUnconnected=off
  wires:
  Current/1 -> O1/1
  Current1/1 -> O2/1
  Current 2/1 -> O3/1
  connections:
  1/RConn1 -- Current/LConn1
  2/RConn1 -- Current/RConn1
  3/RConn1 -- Current1/LConn1
  4/RConn1 -- Current1/RConn1
  5/RConn1 -- Current 2/LConn1
  6/RConn1 -- Current 2/RConn1

== system xieboduoji_13fangzhennow/node3/PV15kW2/Subsystem9 ==
  di : Inport
  Enable : EnablePort
  Pulse tor2 : DiscretePulseGenerator  PulseType=Time based  Period=10e-5  PulseWidth=50
  "integral " : Subsystem  TreatAsAtomicUnit=on
  w : Outport
  wires:
  Pulse tor2/1 -> "integral "/Trigger
  di/1 -> "integral "/1(di)
  "integral "/1(w) -> w/1

== system xieboduoji_13fangzhennow/node3/PV15kW2/改进PLL1 ==
  abc : Inport
  Add : Sum
  Alpha-Beta-Zero to dq0 : powerlib_meascontrol/Transformations/Alpha-Beta-Zero to dq0  Alignment=Aligned with phase A axis
  Constant : Constant  Value=100*pi
  Constant3 : Constant  Value=2*pi
  Demux1 : Demux  Outputs=3
  Gain1 : Gain  Commented=on  Gain=0.5/pi
  Goto2 : Goto  Commented=on  GotoTag=vp
  Integrator : Integrator
  Math Function : Math  Operator=mod  SignedPower=on
  PI : Subsystem  TreatAsAtomicUnit=on
  PID Controller : simulink/Continuous/PID Controller  Controller=P  Form=Parallel  TimeDomain=Discrete-time  UseExternalTs=off  SampleTime=10e-5  IntegratorMethod=Forward Euler  FilterMethod=Forward Euler  ControllerParametersSource=internal  P=1  I=1  D=0  UseFilter=on  N=100  TunerSelectOption=Transfer Function Based (PID Tuner App)  InitialConditionSource=internal  InitialConditionForIntegrator=0  InitialConditionForFilter=0  DifferentiatorICPrevScaledInput=0  ExternalReset=none  TrackingMode=off  Kt=1  LimitOutput=off  UpperSaturationLimit=inf  LowerSaturationLimit=-inf  LinearizeAsGain=on  AntiWindupMode=none  Kb=1  POutMin=[]  POutMax=[]  IOutMin=[]  IOutMax=[]  DOutMin=[]  DOutMax=[]  NOutMin=[]  NOutMax=[]  SumOutMin=[]  SumOutMax=[]  SaturationOutMin=[]  SaturationOutMax=[]  PParamMin=[]  PParamMax=[]  IParamMin=[]  IParamMax=[]  DParamMin=[]  DParamMax=[]  NParamMin=[]  NParamMax=[]  KbParamMin=[]  KbParamMax=[]  KtParamMin=[]  KtParamMax=[]  KbOutMin=[]  KbOutMax=[]  KtOutMin=[]  KtOutMax=[]  IntegratorOutMin=[]  IntegratorOutMax=[]  FilterOutMin=[]  FilterOutMax=[]  SumI1OutMin=[]  SumI1OutMax=[]  SumI2OutMin=[]  SumI2OutMax=[]  SumI3OutMin=[]  SumI3OutMax=[]  SumI4OutMin=[]  SumI4OutMax=[]  SumDOutMin=[]  SumDOutMax=[]  DifferentiatorOutMin=[]  DifferentiatorOutMax=[]  FilterDiffOutCoefMin=[]  FilterDiffOutCoefMax=[]  ReciprocalOutMin=[]  ReciprocalOutMax=[]  SumDenOutMin=[]  SumDenOutMax=[]  SumNumOutMin=[]  SumNumOutMax=[]  DivideOutMin=[]  DivideOutMax=[]  UdiffTsProdOutMin=[]  UdiffTsProdOutMax=[]  NTsProdOutMin=[]  NTsProdOutMax=[]  UintegralTsProdOutMin=[]  UintegralTsProdOutMax=[]  UngainTsProdOutMin=[]  UngainTsProdOutMax=[]  IntegratorContinuousStateAttributes=''  IntegratorStateMustResolveToSignalObject=off  IntegratorRTWStateStorageClass=Auto  FilterContinuousStateAttributes=''  FilterStateMustResolveToSignalObject=off  FilterRTWStateStorageClass=Auto  ParallelPVariant=InternalParameters  IdealPVariant=Disabled  IVariant=Disabled  DVariant=Disabled  IntegratorVariant=Disabled  SatVariant=Disabled  AWVariant=Disabled  PCopyVariant=Disabled  TRVariant=Disabled  FdbkBlocksVariant=Forward  IdealPFdbkVariant=Disabled  SatFdbkVariant=Disabled  DerivativeFilterVariant=Disabled  NVariant=Disabled  NCopyVariant=Disabled_SignalSpec  FilterICVariant=Disabled  IntegratorICVariant=Disabled  ExternalResetVariant=Disabled  TRSumVariant=Passthrough  SumFdbkVariant=Disabled  SumVariant=Passthrough_P  TsampFilterVariant=InternalTs  TsampNgainVariant=Passthrough  TsampIntegralVariant=Disabled_SignalSpec
  Pulse tor2 : DiscretePulseGenerator  PulseType=Time based  Period=5e-5  PulseWidth=50
  Scope : Scope
  Scope1 : Scope  Commented=on
  Scope3 : Scope  Commented=on
  Subsystem2 : Subsystem
  Terminator : Terminator
  abc to Alpha-Beta-Zero1 : powerlib_meascontrol/Transformations/abc to Alpha-Beta-Zero
  mean1 : powerlib_meascontrol/Measurements/Mean  Commented=on  Freq=100  Vinit=0  Ts=10e-5
  mean2 : powerlib_meascontrol/Measurements/Mean  Freq=100  Vinit=0  Ts=10e-5
  Out2 : Outport
  vab0 : Outport  Port=2
  wires:
  Demux1/3 -> Terminator/1
  mean2/1 -> PID Controller/1, PI/1(Vgq)
  abc/1 -> abc to Alpha-Beta-Zero1/1
  mean1/1 -> Scope3/1, Goto2/1
  Demux1/2 -> mean2/1
  Pulse tor2/1 -> PI/Trigger
  PI/1(w) -> Add/2
  Constant/1 -> Add/1
  Alpha-Beta-Zero to dq0/1 -> Demux1/1
  Add/1 -> Gain1/1, Integrator/1
  Math Function/1 -> Out2/1, [wt], Alpha-Beta-Zero to dq0/2
  Constant3/1 -> Math Function/2
  Integrator/1 -> Math Function/1
  Gain1/1 -> Scope1/1
  PID Controller/1 -> Scope/1
  Demux1/1 -> mean1/1
  abc to Alpha-Beta-Zero1/1 -> vab0/1, Subsystem2/1(In1)
  Subsystem2/1(Out1) -> Alpha-Beta-Zero to dq0/1

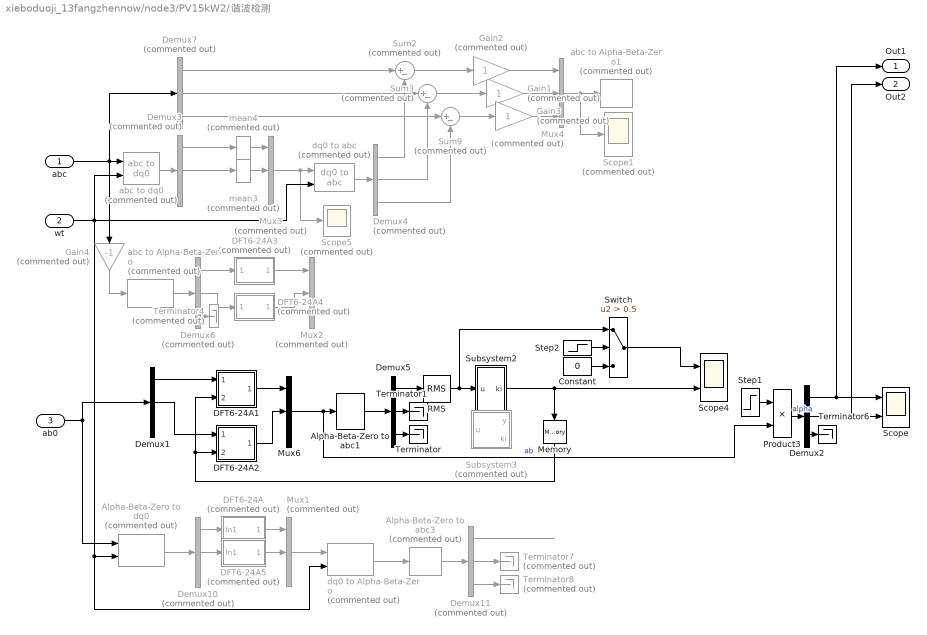
== system xieboduoji_13fangzhennow/node3/PV15kW2/谐波检测 ==
  abc : Inport
  wt : Inport  Port=2
  ab0 : Inport  Port=3
  Alpha-Beta-Zero to abc1 : powerlib_meascontrol/Transformations/Alpha-Beta-Zero to abc
  Alpha-Beta-Zero to abc3 : powerlib_meascontrol/Transformations/Alpha-Beta-Zero to abc  Commented=on
  Alpha-Beta-Zero to dq0 : powerlib_meascontrol/Transformations/Alpha-Beta-Zero to dq0  Commented=on  Alignment=Aligned with phase A axis
  Constant : Constant  Value=0
  DFT6-24A : Subsystem  Commented=on
  DFT6-24A1 : Subsystem
  DFT6-24A2 : Subsystem
  DFT6-24A3 : Subsystem  Commented=on
  DFT6-24A4 : Subsystem  Commented=on
  DFT6-24A5 : Subsystem  Commented=on
  Demux1 : Demux  Outputs=3
  Demux{3..4,6..7,10..11} (6 alike) : Demux  Commented=on  Outputs=3
  Demux2 : Demux  Outputs=3
  Demux5 : Demux  Outputs=3
  Gain1 : Gain  Commented=on
  Gain2 : Gain  Commented=on
  Gain3 : Gain  Commented=on
  Gain4 : Gain  Commented=on  Gain=-1
  Memory : Memory
  Mux{1..4} (4 alike) : Mux  Commented=on  Inputs=3
  Mux6 : Mux  Inputs=3
  Product3 : Product
  RMS : powerlib_meascontrol/Measurements/RMS  TrueRMS=on  Freq=50  RMSInit=0  Ts=5e-5
  Scope : Scope  NumInputPorts=2
  Scope1 : Scope  Commented=on
  Scope4 : Scope  NumInputPorts=2
  Scope5 : Scope  Commented=on
  Step1 : Step  After=-1  SampleTime=0
  Step2 : Step  SampleTime=0
  Subsystem2 : Subsystem
  Subsystem3 : Subsystem  Commented=on
  Sum2 : Sum  Commented=on  Inputs=|+-
  Sum3 : Sum  Commented=on  Inputs=|+-
  Sum9 : Sum  Commented=on  Inputs=|+-
  Switch : Switch  Criteria=u2 > Threshold  Threshold=0.5  SaturateOnIntegerOverflow=off  InputSameDT=off
  Terminator : Terminator
  Terminator1 : Terminator
  Terminator4 : Terminator  Commented=on
  Terminator6 : Terminator
  Terminator7 : Terminator  Commented=on
  Terminator8 : Terminator  Commented=on
  abc to Alpha-Beta-Zero : powerlib_meascontrol/Transformations/abc to Alpha-Beta-Zero  Commented=on
  abc to Alpha-Beta-Zero1 : powerlib_meascontrol/Transformations/abc to Alpha-Beta-Zero  Commented=on
  abc to dq0 : powerlib_meascontrol/Transformations/abc to dq0  Commented=on  Alignment=Aligned with phase A axis
  dq0 to Alpha-Beta-Zero : powerlib_meascontrol/Transformations/dq0 to Alpha-Beta-Zero  Commented=on  Alignment=Aligned with phase A axis
  dq0 to abc : powerlib_meascontrol/Transformations/dq0 to abc  Commented=on  Alignment=Aligned with phase A axis
  mean3 : powerlib_meascontrol/Measurements/Mean  Commented=on  Freq=100  Vinit=0  Ts=5e-5
  mean4 : powerlib_meascontrol/Measurements/Mean  Commented=on  Freq=100  Vinit=0  Ts=5e-5
  Out1 : Outport
  Out2 : Outport  Port=2
  wires:
  Sum2/1 -> Gain2/1
  Mux3/1 -> Scope5/1, dq0 to abc/1
  Demux3/1 -> mean4/1
  wt/1 -> dq0 to abc/2, abc to dq0/2, Alpha-Beta-Zero to dq0/2, dq0 to Alpha-Beta-Zero/2
  Sum9/1 -> Gain3/1
  Demux4/2 -> Sum3/2
  Sum3/1 -> Gain1/1
  mean4/1 -> Mux3/1
  abc to dq0/1 -> Demux3/1
  Demux7/1 -> Sum2/1
  dq0 to abc/1 -> Demux4/1
  Demux4/1 -> Sum2/2
  Demux4/3 -> Sum9/2
  mean3/1 -> Mux3/2
  Demux7/2 -> Sum3/1
  abc/1 -> Demux7/1, Gain4/1, abc to dq0/1
  Demux7/3 -> Sum9/1
  Demux3/2 -> mean3/1
  Mux4/1 -> Scope1/1, abc to Alpha-Beta-Zero1/1
  Product3/1 -> Demux2/1  "alpha"
  Step1/1 -> Product3/1
  Demux1/1 -> DFT6-24A1/1(In1)
  Demux1/2 -> DFT6-24A2/1(In1)
  Alpha-Beta-Zero to abc1/1 -> Demux5/1
  DFT6-24A1/1(Out1) -> Mux6/1
  DFT6-24A2/1(Out1) -> Mux6/2
  Demux5/1 -> RMS/1
  Gain2/1 -> Mux4/1
  Gain1/1 -> Mux4/2
  Gain3/1 -> Mux4/3
  Demux2/1 -> Out1/1, Scope/1
  Demux2/2 -> Out2/1, Scope/2
  abc to Alpha-Beta-Zero/1 -> Demux6/1
  DFT6-24A4/1(Out1) -> Mux2/2
  DFT6-24A3/1(Out1) -> Mux2/1
  Demux6/2 -> DFT6-24A4/1(In1)
  Demux6/1 -> DFT6-24A3/1(In1)
  Demux5/2 -> Terminator1/1
  Demux5/3 -> Terminator/1
  Demux6/3 -> Terminator4/1
  Demux2/3 -> Terminator6/1
  ab0/1 -> Demux1/1, Alpha-Beta-Zero to dq0/1
  Alpha-Beta-Zero to dq0/1 -> Demux10/1
  Demux10/1 -> DFT6-24A/1(In1)
  Demux10/2 -> DFT6-24A5/1(In1)
  DFT6-24A/1(Out1) -> Mux1/1
  DFT6-24A5/1(Out1) -> Mux1/2
  Alpha-Beta-Zero to abc3/1 -> Demux11/1
  Demux11/2 -> Terminator7/1
  Demux11/3 -> Terminator8/1
  Demux11/1 -> ?
  Mux1/1 -> dq0 to Alpha-Beta-Zero/1
  dq0 to Alpha-Beta-Zero/1 -> Alpha-Beta-Zero to abc3/1
  Subsystem2/1(ki) -> Memory/1, Scope4/2
  Step2/1 -> Switch/2
  Constant/1 -> Switch/3
  RMS/1 -> Switch/1, Subsystem2/1(u)
  Switch/1 -> Scope4/1
  Gain4/1 -> abc to Alpha-Beta-Zero/1
  Memory/1 -> DFT6-24A1/2(In2), DFT6-24A2/2(In2)
  Mux6/1 -> Product3/2, Alpha-Beta-Zero to abc1/1  "ab"

== system xieboduoji_13fangzhennow/node3/PV15kW3/PV_Cells2 ==
  note: I0
  note: Iph
  G : Inport
  T : Inport  Port=2
  U : Inport  Port=3
  Add{,3..4,6} (4 alike) : Sum
  Add1 : Sum  Inputs=+-
  Add2 : Sum  Inputs=-+
  Add5 : Sum  Inputs=-+
  Add7 : Sum  Inputs=+-
  C to K : Constant  Value=273.16
  Controlled Current Source : spsControlledCurrentSourceLib/Controlled Current Source  Initialize=on  Source_Type=DC  Amplitude=0  Phase=0  Frequency=0  Measurements=None
  Current Measurement : spsCurrentMeasurementLib/Current Measurement  PhasorSimulation=off  OutputType=Complex  PSBequivalent=0
  Divide{,1..3} (4 alike) : Product  Inputs=*/
  Divide4 : Product  Inputs=**
  Gain : Gain  Gain=1/Series
  Gain1 : Gain  Gain=1/Parallel
  Gn : Constant  Value=1000
  Isc,n : Constant  Value=8.214*Parallel
  Ki : Constant  Value=0.0032*Parallel
  Kv : Constant  Value=-0.123
  Math : Math  SignedPower=on
  Math2 : Math  SignedPower=on
  Nc*K/Q*a : Constant  Value=0.00008629*1.3*54
  Product{,1..4} (5 alike) : Product  RndMeth=Zero
  Rs : Constant  Value=0.221
  Scope : Scope
  Tn : Constant  Value=298.16
  Unit Delay : UnitDelay  SampleTime=-1  HasFrameUpgradeWarning=on
  Voc,n : Constant  Value=32.9
  constant : Constant
  constant2 : Constant
  I_positive : PMIOPort  Tag=PMCPort  Side=Right
  I_negative : PMIOPort  Tag=PMCPort  Port=2  Side=Right
  wires:
  Divide4/1 -> Add6/2  "Rs"
  Divide/1 -> Product/1
  Isc,n/1 -> Add/1
  Product1/1 -> Add/2
  Divide2/1 -> Math/1
  Add/1 -> [I], Product/2
  T/1 -> Add3/1
  Add2/1 -> Divide1/2
  Math/1 -> Add2/2
  [I] -> Divide1/1
  Add1/1 -> [delta_T], Product1/1
  Tn/1 -> Add1/2
  Ki/1 -> Product1/2
  Product/1 -> Add7/1
  Nc*K/Q*a/1 -> Product2/2
  Kv/1 -> Product3/1
  Voc,n/1 -> Add4/2
  Current Measurement/1 -> Unit Delay/1
  [T] -> Product2/1
  [delta_T] -> Product3/2
  Add6/1 -> Divide3/1
  U/1 -> Gain/1
  Rs/1 -> Divide4/1
  Divide1/1 -> Product4/1
  Add7/1 -> Controlled Current Source/1
  Product4/1 -> Add7/2
  constant2/1 -> Add5/1
  Add5/1 -> Product4/2
  [Iout] -> Gain1/1
  Math2/1 -> Scope/1, Add5/2
  Divide3/1 -> Math2/1
  C to K/1 -> Add3/2
  Product2/1 -> Divide3/2, Divide2/2  "Vt*a"
  Add4/1 -> Divide2/1
  Product3/1 -> Add4/1
  Gn/1 -> Divide/2
  constant/1 -> Add2/1
  Add3/1 -> [T], Add1/1
  G/1 -> Divide/1
  Unit Delay/1 -> [Iout]
  Gain/1 -> Add6/1
  Gain1/1 -> Divide4/2
  connections:
  I_negative/RConn1 -- Controlled Current Source/LConn1
  I_positive/RConn1 -- Current Measurement/RConn1
  Controlled Current Source/RConn1 -- Current Measurement/LConn1

== system xieboduoji_13fangzhennow/node3/PV15kW3/PWM2 ==
  Via* : Inport
  Vib* : Inport  Port=2
  Enable : EnablePort
  Alpha-Beta-Zero to abc1 : spsAlphaBetaZerotoabcLib/Alpha-Beta-Zero to abc
      settings: LibrarySourceBlock=|
      | sps_lib/Control/Alpha-Beta-Zero
      | to abc
  Mux1 : Mux  Inputs=3
  PWM3 : Subsystem
  Transport Delay1 : TransportDelay  DelayTime=5e-5
  switch : Outport  PortDimensions=6  VectorParamsAs1DForOutWhenUnconnected=off
  Out1 : Outport  Port=2  VectorParamsAs1DForOutWhenUnconnected=off
  wires:
  Via*/1 -> Mux1/1
  Vib*/1 -> Mux1/2
  Alpha-Beta-Zero to abc1/1 -> PWM3/1(In1)
  PWM3/1(switch) -> switch/1
  PWM3/2(Out1) -> Out1/1
  Mux1/1 -> Alpha-Beta-Zero to abc1/1

== system xieboduoji_13fangzhennow/node3/PV15kW3/Subsystem3 ==
  In2 : Inport
  In1 : Inport  Port=2
  Add1 : Sum  Inputs=+++
  Add3 : Sum  Inputs=+++
  Demux{1..3,5} (4 alike) : Demux  Outputs=3
  Mux1 : Mux  Inputs=3
  Mux2 : Mux  Inputs=3
  Mux3 : Mux  Inputs=3
  Terminator : Terminator
  Transfer Fcn1 : TransferFcn  Numerator=[2.3*3.14*0.9695 -2.3*3.14*600*pi*0.2588]  Denominator=[1 0.7*3.14 360000*pi*pi]
  Transfer Fcn10 : TransferFcn  Commented=on  Numerator=[3.1*3.14 0]  Denominator=[1 0.7*3.14 360000*pi*pi]
  Transfer Fcn11 : TransferFcn  Commented=on  Numerator=[3.1*3.14*0.9695 -3.1*3.14*600*pi*0.2588]  Denominator=[1 0.7*3.14 360000*pi*pi]
  Transfer Fcn12 : TransferFcn  Commented=on  Numerator=[1.2*3.14*0.5 -1.2*3.14*1800*pi*0.866]  Denominator=[1 0.4*3.14 3240000*pi*pi]
  Transfer Fcn13 : TransferFcn  Commented=on  Numerator=[1.2*3.14*0.1736 -1.2*3.14*1800*pi*0.9848]  Denominator=[1 0.4*3.14 3240000*pi*pi]
  Transfer Fcn14 : TransferFcn  Commented=on  Numerator=[1.7*3.14*0.866 -1.7*3.14*1200*pi*0.5]  Denominator=[1 0.5*3.14 1440000*pi*pi]
  Transfer Fcn15 : TransferFcn  Numerator=[0.65*3.14*0.5736 -0.65*3.14*1800*pi*0.81915]  Denominator=[1 0.24*3.14 3240000*pi*pi]
  Transfer Fcn16 : TransferFcn  Commented=on  Numerator=[3.2*3.14 0]  Denominator=[1 0.7*3.14 360000*pi*pi]
  Transfer Fcn17 : TransferFcn  Commented=on  Numerator=[0.65*3.14*0.5736 -0.65*3.14*1800*pi*0.81915]  Denominator=[1 0.24*3.14 3240000*pi*pi]
  Transfer Fcn19 : TransferFcn  Commented=on  Numerator=[1.9*3.14*0.9703 -1.9*3.14*1200*pi*0.2419]  Denominator=[1 0.55*3.14 1440000*pi*pi]
  Transfer Fcn2 : TransferFcn  Numerator=[1.7*3.14*0.866 -1.7*3.14*1200*pi*0.5]  Denominator=[1 0.5*3.14 1440000*pi*pi]
  Transfer Fcn20 : TransferFcn  Commented=on  Numerator=[0.7*3.14*0.707 -0.7*3.14*1800*pi*0.707]  Denominator=[1 0.25*3.14 3240000*pi*pi]
  Transfer Fcn3 : TransferFcn  Numerator=[0.65*3.14*0.707 -0.65*3.14*1800*pi*0.707]  Denominator=[1 0.24*3.14 3240000*pi*pi]
  Transfer Fcn4 : TransferFcn  Numerator=[2.3*3.14*0.9695 -2.3*3.14*600*pi*0.2588]  Denominator=[1 0.7*3.14 360000*pi*pi]
  Transfer Fcn5 : TransferFcn  Commented=on  Numerator=[0.7*3.14*0.707 -0.7*3.14*1800*pi*0.707]  Denominator=[1 0.25*3.14 3240000*pi*pi]
  Transfer Fcn6 : TransferFcn  Commented=on  Numerator=[0.7*3.14*0.5736 -0.7*3.14*1800*pi*0.81915]  Denominator=[1 0.25*3.14 3240000*pi*pi]
  Transfer Fcn7 : TransferFcn  Commented=on  Numerator=[1.9*3.14*0.766 -1.9*3.14*1200*pi*0.643]  Denominator=[1 0.55*3.14 1440000*pi*pi]
  Transfer Fcn8 : TransferFcn  Numerator=[1.7*3.14*0.866 -1.7*3.14*1200*pi*0.5]  Denominator=[1 0.5*3.14 1440000*pi*pi]
  Transfer Fcn9 : TransferFcn  Numerator=[0.65*3.14*0.707 -0.65*3.14*1800*pi*0.707]  Denominator=[1 0.24*3.14 3240000*pi*pi]
  dq0 to Alpha-Beta-Zero : spsdq0toAlphaBetaZeroLib/dq0 to Alpha-Beta-Zero  Alignment=90 degrees behind phase A axis
  dq0 to Alpha-Beta-Zero1 : spsdq0toAlphaBetaZeroLib/dq0 to Alpha-Beta-Zero  Alignment=90 degrees behind phase A axis
  dq0 to Alpha-Beta-Zero2 : spsdq0toAlphaBetaZeroLib/dq0 to Alpha-Beta-Zero  Alignment=90 degrees behind phase A axis
  Out3 : Outport
  Out1 : Outport  Port=2
  wires:
  In2/1 -> Demux5/1
  Demux5/1 -> Transfer Fcn4/1, Transfer Fcn3/1, Transfer Fcn2/1
  Transfer Fcn4/1 -> Mux1/1
  Transfer Fcn1/1 -> Mux1/2
  Mux1/1 -> dq0 to Alpha-Beta-Zero/1
  dq0 to Alpha-Beta-Zero/1 -> Demux1/1
  Demux1/1 -> Add1/1
  Demux1/2 -> Add3/1
  Add1/1 -> Out3/1
  Add3/1 -> Out1/1
  dq0 to Alpha-Beta-Zero1/1 -> Demux2/1
  Mux2/1 -> dq0 to Alpha-Beta-Zero1/1
  Transfer Fcn8/1 -> Mux2/2
  Transfer Fcn2/1 -> Mux2/1
  Demux2/1 -> Add1/2
  Demux2/2 -> Add3/2
  Demux3/2 -> Add3/3
  Demux3/1 -> Add1/3
  Transfer Fcn3/1 -> Mux3/1
  Transfer Fcn9/1 -> Mux3/2
  Mux3/1 -> dq0 to Alpha-Beta-Zero2/1
  dq0 to Alpha-Beta-Zero2/1 -> Demux3/1
  Demux5/2 -> Transfer Fcn1/1, Transfer Fcn9/1, Transfer Fcn8/1
  In1/1 -> dq0 to Alpha-Beta-Zero1/2, dq0 to Alpha-Beta-Zero2/2, dq0 to Alpha-Beta-Zero/2
  Demux5/3 -> Terminator/1

== system xieboduoji_13fangzhennow/node3/PV15kW3/Subsystem7 ==
  Voltage : spsVoltageMeasurementLib/Voltage Measurement  PhasorSimulation=off  OutputType=Complex  PSBequivalent=0
  Voltage1 : spsVoltageMeasurementLib/Voltage Measurement  PhasorSimulation=off  OutputType=Complex  PSBequivalent=0
  Voltage2 : spsVoltageMeasurementLib/Voltage Measurement  PhasorSimulation=off  OutputType=Complex  PSBequivalent=0
  1 : PMIOPort  Side=Left
  2 : PMIOPort  Port=2  Side=Left
  3 : PMIOPort  Port=3  Side=Left
  4 : PMIOPort  Port=4  Side=Left
  5 : PMIOPort  Port=5  Side=Left
  6 : PMIOPort  Port=6  Side=Left
  O1 : Outport  VectorParamsAs1DForOutWhenUnconnected=off
  O2 : Outport  Port=2  VectorParamsAs1DForOutWhenUnconnected=off
  O3 : Outport  Port=3  VectorParamsAs1DForOutWhenUnconnected=off
  wires:
  Voltage2/1 -> O3/1
  Voltage1/1 -> O2/1
  Voltage/1 -> O1/1
  connections:
  6/RConn1 -- Voltage2/LConn2
  5/RConn1 -- Voltage2/LConn1
  4/RConn1 -- Voltage1/LConn2
  3/RConn1 -- Voltage1/LConn1
  2/RConn1 -- Voltage/LConn2
  1/RConn1 -- Voltage/LConn1

== system xieboduoji_13fangzhennow/node3/PV15kW3/Subsystem8 ==
  Current : spsCurrentMeasurementLib/Current Measurement  PhasorSimulation=off  OutputType=Complex  PSBequivalent=0
  Current 2 : spsCurrentMeasurementLib/Current Measurement  PhasorSimulation=off  OutputType=Complex  PSBequivalent=0
  Current1 : spsCurrentMeasurementLib/Current Measurement  PhasorSimulation=off  OutputType=Complex  PSBequivalent=0
  1 : PMIOPort  Side=Left
  2 : PMIOPort  Port=2  Side=Right
  3 : PMIOPort  Port=3  Side=Left
  4 : PMIOPort  Port=4  Side=Right
  5 : PMIOPort  Port=5  Side=Left
  6 : PMIOPort  Port=6  Side=Right
  O1 : Outport  VectorParamsAs1DForOutWhenUnconnected=off
  O2 : Outport  Port=2  VectorParamsAs1DForOutWhenUnconnected=off
  O3 : Outport  Port=3  VectorParamsAs1DForOutWhenUnconnected=off
  wires:
  Current/1 -> O1/1
  Current1/1 -> O2/1
  Current 2/1 -> O3/1
  connections:
  1/RConn1 -- Current/LConn1
  2/RConn1 -- Current/RConn1
  3/RConn1 -- Current1/LConn1
  4/RConn1 -- Current1/RConn1
  5/RConn1 -- Current 2/LConn1
  6/RConn1 -- Current 2/RConn1

== system xieboduoji_13fangzhennow/node3/PV15kW3/Subsystem9 ==
  di : Inport
  Enable : EnablePort
  Pulse tor2 : DiscretePulseGenerator  PulseType=Time based  Period=10e-5  PulseWidth=50
  "integral " : Subsystem  TreatAsAtomicUnit=on
  w : Outport
  wires:
  Pulse tor2/1 -> "integral "/Trigger
  di/1 -> "integral "/1(di)
  "integral "/1(w) -> w/1

== system xieboduoji_13fangzhennow/node3/PV15kW3/改进PLL1 ==
  abc : Inport
  Add : Sum
  Alpha-Beta-Zero to dq0 : spsAlphaBetaZerotodq0Lib/Alpha-Beta-Zero to dq0  Alignment=Aligned with phase A axis
  Constant : Constant  Value=100*pi
  Constant3 : Constant  Value=2*pi
  Demux1 : Demux  Outputs=3
  Gain1 : Gain  Commented=on  Gain=0.5/pi
  Goto2 : Goto  Commented=on  GotoTag=vp
  Integrator : Integrator
  Math Function : Math  Operator=mod  SignedPower=on
  PI : Subsystem  TreatAsAtomicUnit=on
  PID Controller : slpidlib/PID Controller  Controller=P  Form=Parallel  TimeDomain=Discrete-time  UseExternalTs=off  SampleTime=10e-5  IntegratorMethod=Forward Euler  FilterMethod=Forward Euler  ControllerParametersSource=internal  P=1  I=1  UseKiTs=off  D=0  N=100  UseFilter=on  TunerSelectOption=Transfer Function Based (PID Tuner App)  InitialConditionSource=internal  InitialConditionForIntegrator=0  InitialConditionForFilter=0  DifferentiatorICPrevScaledInput=0  ExternalReset=none  TrackingMode=off  Kt=1  LimitOutput=off  SatLimitsSource=internal  UpperSaturationLimit=inf  LowerSaturationLimit=-inf  LinearizeAsGain=on  AntiWindupMode=none  Kb=1  LimitIntegrator=off  UpperIntegratorSaturationLimit=inf  LowerIntegratorSaturationLimit=-inf  POutMin=[]  POutMax=[]  IOutMin=[]  IOutMax=[]  DOutMin=[]  DOutMax=[]  NOutMin=[]  NOutMax=[]  SumOutMin=[]  SumOutMax=[]  SaturationOutMin=[]  SaturationOutMax=[]  PParamMin=[]  PParamMax=[]  IParamMin=[]  IParamMax=[]  DParamMin=[]  DParamMax=[]  NParamMin=[]  NParamMax=[]  KbParamMin=[]  KbParamMax=[]  KtParamMin=[]  KtParamMax=[]  KbOutMin=[]  KbOutMax=[]  KtOutMin=[]  KtOutMax=[]  IntegratorOutMin=[]  IntegratorOutMax=[]  FilterOutMin=[]  FilterOutMax=[]  SumI1OutMin=[]  SumI1OutMax=[]  SumI2OutMin=[]  SumI2OutMax=[]  SumI3OutMin=[]  SumI3OutMax=[]  SumI4OutMin=[]  SumI4OutMax=[]  SumDOutMin=[]  SumDOutMax=[]  DifferentiatorOutMin=[]  DifferentiatorOutMax=[]  FilterDiffOutCoefMin=[]  FilterDiffOutCoefMax=[]  ReciprocalOutMin=[]  ReciprocalOutMax=[]  SumDenOutMin=[]  SumDenOutMax=[]  SumNumOutMin=[]  SumNumOutMax=[]  DivideOutMin=[]  DivideOutMax=[]  UdiffTsProdOutMin=[]  UdiffTsProdOutMax=[]  NTsProdOutMin=[]  NTsProdOutMax=[]  UintegralTsProdOutMin=[]  UintegralTsProdOutMax=[]  UngainTsProdOutMin=[]  UngainTsProdOutMax=[]  ClampingZeroOutDataTypeStr=Inherit: Inherit via back propagation  ClampingZeroOutMin=[]  ClampingZeroOutMax=[]  FilterDenConstantOutDataTypeStr=Inherit: Inherit via back propagation  FilterDenConstantOutMin=[]  FilterDenConstantOutMax=[]  PCopyOutDataTypeStr=Inherit: Inherit via back propagation  PCopyOutMin=[]  PCopyOutMax=[]  NCopyOutDataTypeStr=Inherit: Inherit via back propagation  NCopyOutMin=[]  NCopyOutMax=[]  IntegratorContinuousStateAttributes=''  IntegratorStateMustResolveToSignalObject=off  IntegratorRTWStateStorageClass=Auto  FilterContinuousStateAttributes=''  FilterStateMustResolveToSignalObject=off  FilterRTWStateStorageClass=Auto  ParallelPVariant=InternalParameters  IdealPVariant=Disabled  IVariant=Disabled  DVariant=Disabled  IntegratorVariant=Disabled  SatVariant=Disabled  AWVariant=Disabled  PCopyVariant=Disabled  TRVariant=Disabled  FdbkBlocksVariant=Forward  IdealPFdbkVariant=Disabled  SatFdbkVariant=Disabled  DerivativeFilterVariant=Disabled  NVariant=Disabled  NCopyVariant=Disabled_SignalSpec  FilterICVariant=Disabled  IntegratorICVariant=Disabled  ExternalResetVariant=Disabled  TRSumVariant=Passthrough  SumFdbkVariant=Disabled  SumVariant=Passthrough_P  TsampFilterVariant=InternalTs  TsampNgainVariant=Passthrough  TsampIntegralVariant=Disabled_SignalSpec  ExternalSaturationOutDataTypeStr=Inherit: Same as second input
  Pulse tor2 : DiscretePulseGenerator  PulseType=Time based  Period=5e-5  PulseWidth=50
  Scope : Scope
  Scope1 : Scope  Commented=on
  Scope2 : Scope
  Scope3 : Scope  Commented=on
  Scope4 : Scope
  Subsystem2 : Subsystem
  Sum : Sum  Inputs=|+-
  Terminator : Terminator
  abc to Alpha-Beta-Zero1 : spsabctoAlphaBetaZeroLib/abc to Alpha-Beta-Zero
  mean1 : spsMeanLib/Mean  Commented=on  Freq=100  Vinit=0  Ts=10e-5
  mean2 : spsMeanLib/Mean  Freq=100  Vinit=0  Ts=5e-5
  Out2 : Outport
  vab0 : Outport  Port=2
  wires:
  Demux1/3 -> Terminator/1
  mean2/1 -> PID Controller/1, PI/1(Vgq)
  abc/1 -> abc to Alpha-Beta-Zero1/1
  mean1/1 -> Scope3/1, Goto2/1
  Demux1/2 -> mean2/1
  Pulse tor2/1 -> PI/Trigger
  PI/1(w) -> Add/2
  Constant/1 -> Add/1
  Alpha-Beta-Zero to dq0/1 -> Demux1/1
  Add/1 -> Gain1/1, Integrator/1
  Math Function/1 -> Out2/1, Scope4/1, [wt], Alpha-Beta-Zero to dq0/2
  Constant3/1 -> Math Function/2
  Integrator/1 -> Math Function/1
  Gain1/1 -> Scope1/1
  PID Controller/1 -> Scope/1
  Demux1/1 -> mean1/1
  abc to Alpha-Beta-Zero1/1 -> Sum/1, Subsystem2/1(In1)
  Subsystem2/1(vab0) -> Alpha-Beta-Zero to dq0/1, Sum/2
  Sum/1 -> Scope2/1, vab0/1
